simulink model "HDLRxDemodulator"  (R2024a)
settings: Solver=FixedStepDiscrete  StartTime=0.0  StopTime=stopTime  RelTol=1e-3
model workspace (MAT data in the model file):
  HDLVAXIManagerConfig = hdlverifier.internal.AXIMaster.ConfigParams
values from neighbouring files (symbols this model uses):
  payloadBitsPerSubcarrier = binl2dec(batId)    [parameters.m]
  payloadCyclicPrefixLen = binl2dec(cyclicPrefixId) * N / 32    [parameters.m]
  psduSizeLSB = flip(psduSize)    [testRxDemodulator.m]
undefined symbols (not defined in the file or in its folder): fPHY, fs
libraries: HDL_ieee_8021513 x3, dspsrcs4 x2, whdlutilities x2
settings Model: DataTypeOverride=Off  SimulationMode=accelerator  Creator=cotti  LastModifiedBy=cotti
settings OptimizationCC: BlockReduction=off  ConditionallyExecuteInputs=off  DefaultParameterBehavior=Inlined  InheritOutputTypeSmallerThanSingle=on
settings DebuggingCC: ArtificialAlgebraicLoopMsg=error  SingleTaskRateTransMsg=error
settings HardwareCC: ProdBitPerPointer=32  ProdBitPerSizeT=32  ProdBitPerPtrDiffT=32  ProdLargestAtomicFloat=None  ProdIntDivRoundTo=Undefined  ProdEndianess=Unspecified  ProdWordSize=32  ProdHWDeviceType=ASIC/FPGA->ASIC/FPGA  TargetBitPerLong=64  TargetBitPerPointer=64  TargetBitPerSizeT=64  TargetBitPerPtrDiffT=64  TargetLongLongMode=on  TargetIntDivRoundTo=Zero  TargetEndianess=LittleEndian  TargetWordSize=64  TargetHWDeviceType=Custom Processor->MATLAB Host Computer  ProdEqTarget=off

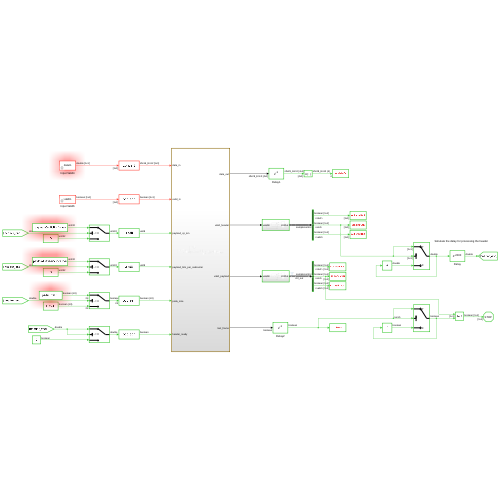
[thumbnail: Simulink's stored preview of the top-level diagram]
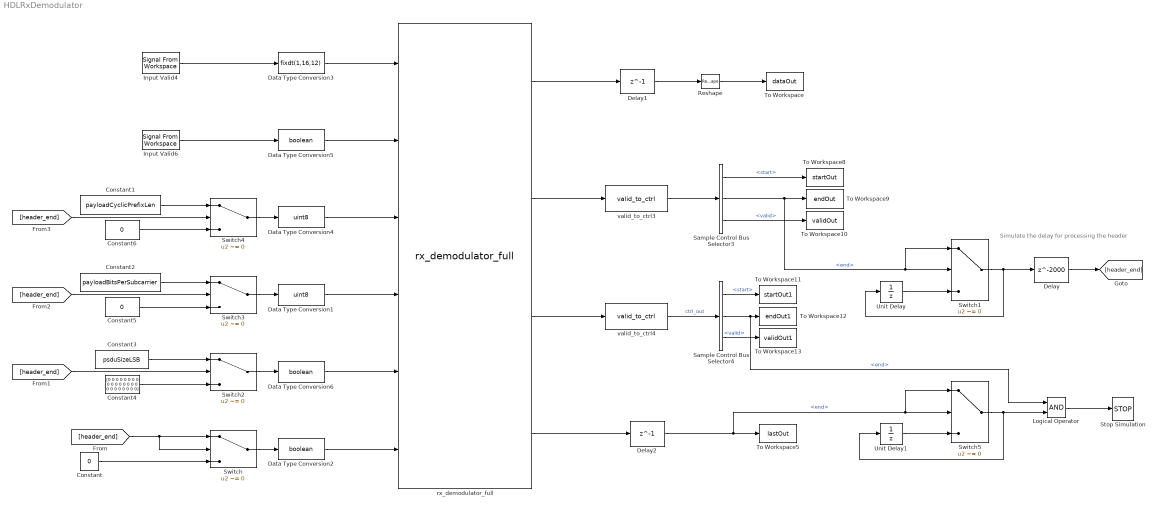
== system HDLRxDemodulator ==
  note: Simulate the delay for processing the header
  Constant : Constant  Value=0  OutDataTypeStr=boolean  SampleTime=1/fPHY
  Constant1 : Constant  Value=payloadCyclicPrefixLen  SampleTime=1/fPHY
  Constant2 : Constant  Value=payloadBitsPerSubcarrier  SampleTime=1/fPHY
  Constant3 : Constant  Value=psduSizeLSB  SampleTime=1/fPHY
  Constant4 : Constant  Value=[0 0 0 0 0 0 0 0 0 0 0 0 0 0 0 0 0 0 0 0 0 0 0 0]  OutDataTypeStr=boolean  SampleTime=1/fPHY
  Constant5 : Constant  Value=0  OutDataTypeStr=uint32  SampleTime=1/fPHY
  Constant6 : Constant  Value=0  OutDataTypeStr=uint32  SampleTime=1/fPHY
  Data Type Conversion1 : DataTypeConversion  OutDataTypeStr=uint8  SaturateOnIntegerOverflow=off  RndMeth=Floor
  Data Type Conversion2 : DataTypeConversion  OutDataTypeStr=boolean  SaturateOnIntegerOverflow=off  RndMeth=Floor
  Data Type Conversion3 : DataTypeConversion  OutDataTypeStr=fixdt(1,16,12)  SaturateOnIntegerOverflow=off  RndMeth=Floor
  Data Type Conversion4 : DataTypeConversion  OutDataTypeStr=uint8  SaturateOnIntegerOverflow=off  RndMeth=Floor
  Data Type Conversion5 : DataTypeConversion  OutDataTypeStr=boolean  SaturateOnIntegerOverflow=off  RndMeth=Floor
  Data Type Conversion6 : DataTypeConversion  OutDataTypeStr=boolean  SaturateOnIntegerOverflow=off  RndMeth=Floor
  Delay : Delay  DelayLength=2000  InitialCondition=0  UseCircularBuffer=on
  Delay1 : Delay  DelayLength=1  InitialCondition=0  UseCircularBuffer=on
  Delay2 : Delay  DelayLength=1  InitialCondition=0  UseCircularBuffer=on
  Input Valid4 : dspsrcs4/Signal From Workspace  X=dataIn  Ts=1/fs  nsamps=1  OutputAfterFinalValue=Cyclic repetition  ignoreOrWarnInputAndFrameLengths=off  OutputFrames=off
  Input Valid6 : dspsrcs4/Signal From Workspace  X=validIn  Ts=1/fs  nsamps=1  OutputAfterFinalValue=Setting to zero  ignoreOrWarnInputAndFrameLengths=off  OutputFrames=off
  Logical Operator : Logic  AllPortsSameDT=off  OutDataTypeStr=boolean
  Reshape : Reshape
  Sample Control Bus Selector3 : whdlutilities/Sample Control Bus Selector  OutputSignals=start,end,valid
  Sample Control Bus Selector4 : whdlutilities/Sample Control Bus Selector  OutputSignals=start,end,valid
  Stop Simulation : Stop
  Switch{,1..5} (6 alike) : Switch  Criteria=u2 ~= 0  SaturateOnIntegerOverflow=off  InputSameDT=off
  To Workspace : ToWorkspace  VariableName=dataOut  SampleTime=1/fPHY
      settings: Save2DSignal=2-D array (concatenate along first dimension)
  To Workspace10 : ToWorkspace  VariableName=validOut  SampleTime=1/fPHY
      settings: Save2DSignal=2-D array (concatenate along first dimension)
  To Workspace11 : ToWorkspace  VariableName=startOut1  SampleTime=1/fPHY
      settings: Save2DSignal=2-D array (concatenate along first dimension)
  To Workspace12 : ToWorkspace  VariableName=endOut1  SampleTime=1/fPHY
      settings: Save2DSignal=2-D array (concatenate along first dimension)
  To Workspace13 : ToWorkspace  VariableName=validOut1  SampleTime=1/fPHY
      settings: Save2DSignal=2-D array (concatenate along first dimension)
  To Workspace5 : ToWorkspace  VariableName=lastOut  SampleTime=1/fPHY
      settings: Save2DSignal=2-D array (concatenate along first dimension)
  To Workspace8 : ToWorkspace  VariableName=startOut  SampleTime=1/fPHY
      settings: Save2DSignal=2-D array (concatenate along first dimension)
  To Workspace9 : ToWorkspace  VariableName=endOut  SampleTime=1/fPHY
      settings: Save2DSignal=2-D array (concatenate along first dimension)
  Unit Delay : UnitDelay  SampleTime=-1  HasFrameUpgradeWarning=on
  Unit Delay1 : UnitDelay  SampleTime=-1  HasFrameUpgradeWarning=on
  rx_demodulator_full : HDL_ieee_8021513/rx_demodulator_full  SystemSampleTime=-1  VariantActivationTime=update diagram  AllowFlexibleInterface=on  Latency=0  AutoFrameSizeCalculation=off
      settings: SourceProductName=HDL IEEE 8021513
  valid_to_ctrl3 : HDL_ieee_8021513/valid_to_ctrl  SystemSampleTime=-1  VariantActivationTime=update diagram  AllowFlexibleInterface=on  Latency=0  AutoFrameSizeCalculation=off
      settings: SourceProductName=HDL IEEE 8021513
  valid_to_ctrl4 : HDL_ieee_8021513/valid_to_ctrl  SystemSampleTime=-1  VariantActivationTime=update diagram  AllowFlexibleInterface=on  Latency=0  AutoFrameSizeCalculation=off
      settings: SourceProductName=HDL IEEE 8021513
  wires:
  Input Valid4/1 -> Data Type Conversion3/1
  Data Type Conversion3/1 -> rx_demodulator_full/1
  Input Valid6/1 -> Data Type Conversion5/1
  Data Type Conversion1/1 -> rx_demodulator_full/4
  Data Type Conversion4/1 -> rx_demodulator_full/3
  Data Type Conversion5/1 -> rx_demodulator_full/2
  Data Type Conversion6/1 -> rx_demodulator_full/5
  rx_demodulator_full/1 -> Delay1/1
  Delay1/1 -> Reshape/1
  rx_demodulator_full/4 -> Delay2/1
  rx_demodulator_full/2 -> valid_to_ctrl3/1
  Sample Control Bus Selector3/1 -> To Workspace8/1  "<start>"
  Sample Control Bus Selector3/2 -> Switch1/1, Switch1/2, To Workspace9/1  "<end>"
  Sample Control Bus Selector3/3 -> To Workspace10/1  "<valid>"
  valid_to_ctrl3/1 -> Sample Control Bus Selector3/1
  rx_demodulator_full/3 -> valid_to_ctrl4/1
  Sample Control Bus Selector4/1 -> To Workspace11/1  "<start>"
  Sample Control Bus Selector4/2 -> Logical Operator/1, To Workspace12/1  "<end>"
  Sample Control Bus Selector4/3 -> To Workspace13/1  "<valid>"
  valid_to_ctrl4/1 -> Sample Control Bus Selector4/1  "ctrl_out"
  Reshape/1 -> To Workspace/1
  Constant/1 -> Switch/3
  [header_end] -> Switch/2, Switch/1
  Unit Delay/1 -> Switch1/3
  Switch1/1 -> Delay/1, Unit Delay/1
  Delay/1 -> [header_end]
  Switch/1 -> Data Type Conversion2/1
  Data Type Conversion2/1 -> rx_demodulator_full/6
  Switch2/1 -> Data Type Conversion6/1
  Switch3/1 -> Data Type Conversion1/1
  Switch4/1 -> Data Type Conversion4/1
  Constant5/1 -> Switch3/3
  Constant4/1 -> Switch2/3
  Constant6/1 -> Switch4/3
  Constant1/1 -> Switch4/1
  Constant2/1 -> Switch3/1
  Constant3/1 -> Switch2/1
  [header_end] -> Switch2/2
  [header_end] -> Switch3/2
  [header_end] -> Switch4/2
  Unit Delay1/1 -> Switch5/3
  Switch5/1 -> Logical Operator/2, Unit Delay1/1
  Delay2/1 -> Switch5/1, Switch5/2, To Workspace5/1  "<end>"
  Logical Operator/1 -> Stop Simulation/1
